simulink model "Q3G1block"  (R2020b)
settings: Solver=VariableStepAuto  StartTime=0.0  StopTime=100  RelTol=1e-3
libraries: cstblocks x5
settings Model: Creator=47845  LastModifiedBy=47845

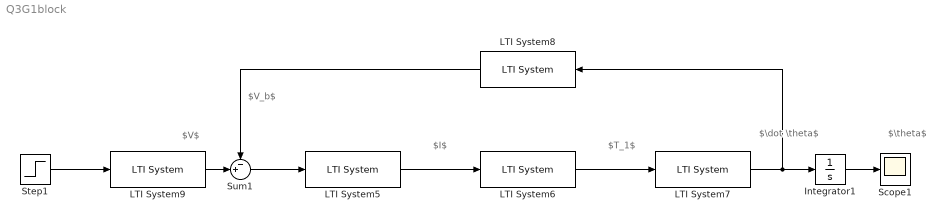
== system Q3G1block ==
  note: $I$
  note: $T_1$
  note: $V_b$
  note: $\theta$
  note: $\dot \theta$
  note: $V$
  Integrator1 : Integrator
  LTI System5 : cstblocks/LTI System  sys=G3  IC=[]
  LTI System6 : cstblocks/LTI System  sys=G4  IC=[]
  LTI System7 : cstblocks/LTI System  sys=G5  IC=[]
  LTI System8 : cstblocks/LTI System  sys=G6  IC=[]
  LTI System9 : cstblocks/LTI System  sys=G1  IC=[]
  Scope1 : Scope
  Step1 : Step  Time=0  SampleTime=0
  Sum1 : Sum  Inputs=-+|
  wires:
  LTI System9/1 -> Sum1/2
  Step1/1 -> LTI System9/1
  Integrator1/1 -> Scope1/1
  LTI System6/1 -> LTI System7/1
  LTI System5/1 -> LTI System6/1
  LTI System8/1 -> Sum1/1
  Sum1/1 -> LTI System5/1
  LTI System7/1 -> Integrator1/1, LTI System8/1
